simulink library "mylibrary"  (Simulink 3.00)
libraries: mathlib x6

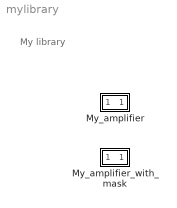
== system mylibrary ==
  note: My library
  My_amplifier : Subsystem
      mask Type: REX sequence
  My_amplifier_with_mask : Subsystem  mask(REX sequence){user_gain=2, user_offset=6}
      mask prompts: user_gain "Amplifier gain"; user_offset "Amplifier offset"

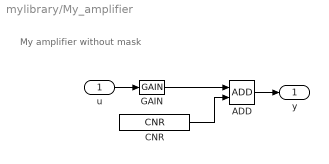
== system mylibrary/My_amplifier ==
  note: My amplifier without mask
  u : Inport  Port=1
  ADD : mathlib/ADD
  CNR : mathlib/CNR  ycn=5
  GAIN : mathlib/GAIN  k=3
  y : Outport  Port=1
  wires:
  ADD/1 -> y/1
  CNR/1 -> ADD/2
  GAIN/1 -> ADD/1
  u/1 -> GAIN/1

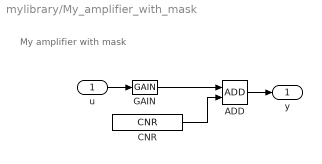
== system mylibrary/My_amplifier_with_mask ==
  note: My amplifier with mask
  u : Inport  Port=1
  ADD : mathlib/ADD
  CNR : mathlib/CNR  ycn=user_offset
  GAIN : mathlib/GAIN  k=user_gain
  y : Outport  Port=1
  wires:
  ADD/1 -> y/1
  CNR/1 -> ADD/2
  GAIN/1 -> ADD/1
  u/1 -> GAIN/1
